simulink model "CicInterpolator75"  (Simulink 6.3)
settings: Solver=VariableStepDiscrete  SolverMode=SingleTasking  StartTime=0.0  StopTime=7000  FixedStep=1  RelTol=1e-3
InitFcn:
  | %% DSPBuilder Start
  | alt_dspbuilder_update_model(bdroot)
  | %% DSPBuilder End
libraries: allblocks_alteradspbuilder2 x15
settings Model: Creator=mjervis  LastModifiedBy=LKONG
settings DataIOCC: SignalLoggingName=sigsOut
settings OptimizationCC: BooleanDataType=off  InlineInvariantSignals=on
settings DebuggingCC: SolverPrmCheckMsg=none
settings HardwareCC: TargetUnknown=on

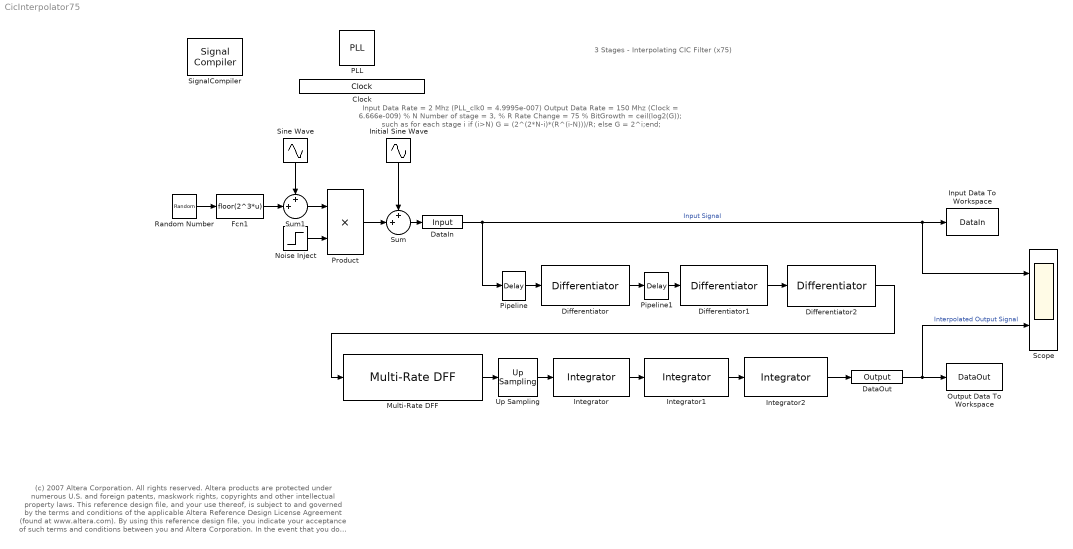
== system CicInterpolator75 ==
  note: 3 Stages - Interpolating CIC Filter (x75)
  note: (c) 2007 Altera Corporation. All rights reserved.  Altera products are protected under numerous U.S. and foreign patents, maskwork rights, copyrights and other intellectual property laws.
      | This reference design file, and your use thereof, is subject to and governed by the terms and conditions of the applicable Altera Reference Design License Agreement (found at www.altera.com).
      | By using this reference design file, you indicate your acceptance of such terms and conditions between you and Altera Corporation.
      | In the event that you do not agree with such terms and conditions, you may not use the reference design file and please promptly destroy any copies you have made.
      | This reference design file being provided on an "as-is" basis and as an accommodation and therefore all warranties, representations or guarantees of any kind (whether express, implied or statutory)
      | including, without limitation, warranties of merchantability, non-infringement, or fitness for a particular purpose, are specifically disclaimed.
      | By making this reference design file available, Altera expressly does not recommend, suggest or require that this reference design file be used in combination with any other product not provided by Altera
  note: Input Data Rate    = 2 Mhz (PLL_clk0 = 4.9995e-007)
      | Output Data Rate = 150 Mhz (Clock   = 6.666e-009)
      |
      | % N Number of stage = 3,
      | % R Rate Change = 75
      | % BitGrowth = ceil(log2(G)); such as for each stage i
      |      if (i>N)     G = (2^(2*N-i)*(R^(i-N)))/R;
      |      else         G = 2^i;end;
  Clock : allblocks_alteradspbuilder2/Clock  ClockPeriod=20/3  ClockPeriodUnit=ns  SampleTime=1  SimulationStartCycle=5  PhaseOffset=0  Reset=aclr  ResetType=Active Low  Export=off
  DataIn : allblocks_alteradspbuilder2/Input  iofile=d:\wsTrunk\workspace\Documentation\DesignExamples\Demos\Filters\CicFilter\Interpolator\tb_CicInterpolator75\CicInterpolator75_DataIn.salt  BusType=Signed Integer  bwl=8  bwr=0  SpecifyClock=on  clock=PLL_clk0  PORTTYPE=Input
  DataOut : allblocks_alteradspbuilder2/Output  iofile=d:\wsTrunk\workspace\Documentation\DesignExamples\Demos\Filters\CicFilter\Interpolator\tb_CicInterpolator75\CicInterpolator75_DataOut.capture  BusType=Signed Integer  bwl=29  bwr=0  PORTTYPE=Output
  Differentiator : allblocks_alteradspbuilder2/Differentiator  bwl=29  depth=1  use_ena=off  use_sclr=off
  Differentiator1 : allblocks_alteradspbuilder2/Differentiator  bwl=29  depth=1  use_ena=off  use_sclr=off
  Differentiator2 : allblocks_alteradspbuilder2/Differentiator  bwl=29  depth=1  use_ena=off  use_sclr=off
  Fcn1 : Fcn  Expr=floor(2^3*u)
  Initial Sine Wave : Sin  Orientation=down  SineType=Sample based  Amplitude=2^6 -1  SampleTime=75
  Input Data To Workspace : ToWorkspace  VariableName=DataIn  SampleTime=-1  SaveFormat=Array
  Integrator : allblocks_alteradspbuilder2/Integrator  bwl=29  depth=1  use_ena=off  use_sclr=off
  Integrator1 : allblocks_alteradspbuilder2/Integrator  bwl=29  depth=1  use_ena=off  use_sclr=off
  Integrator2 : allblocks_alteradspbuilder2/Integrator  bwl=29  depth=1  use_ena=off  use_sclr=off
  Multi-Rate DFF : allblocks_alteradspbuilder2/Multi-Rate DFF  pipeline=1  UseBaseClock=off  clock=Clock  use_ena=off  use_sclr=off
  Noise Inject : Step  Time=2500  SampleTime=75
  Output Data To Workspace : ToWorkspace  VariableName=DataOut  SampleTime=-1  SaveFormat=Array
  PLL : allblocks_alteradspbuilder2/PLL  clock_mult=[75, 75, 3, 4, 1, 1, 1, 1, 1]  clock_divide=[1, 1, 3, 1, 1, 1, 1, 1, 1]  clock_export=[0, 0, 0, 0, 0, 0, 0, 0, 0]  num_clocks=1  input_clock=Clock  use_base_clock=on
  Pipeline : allblocks_alteradspbuilder2/Delay  pipeline=1  ClockPhase=1  use_ena=off  use_sclr=off  use_init=off  reset_value=1
  Pipeline1 : allblocks_alteradspbuilder2/Delay  pipeline=1  ClockPhase=1  use_ena=off  use_sclr=off  use_init=off  reset_value=1
  Product : Product  SaturateOnIntegerOverflow=on  InputSameDT=on
  Random Number : RandomNumber  Variance=8  SampleTime=75
  Scope : Scope  NumInputPorts=2
      settings: TimeRange=7000  YMin=-100~-600000  YMax=150~600000  MaxDataPoints=10000
  SignalCompiler : allblocks_alteradspbuilder2/Signal Compiler  DeviceFamily=Stratix III  DeviceName=AUTO  EnableSignalTap=off  SignalTapDepth=128  UseBoardBlock=off  StpUseDefaultClock=on  StpClock=clock
  Sine Wave : Sin  Orientation=down  SineType=Sample based  Amplitude=2^3 -1  Samples=500  SampleTime=75
  Sum : Sum  Inputs=++|  SaturateOnIntegerOverflow=on  InputSameDT=on
  Sum1 : Sum  Inputs=++|  SaturateOnIntegerOverflow=on  InputSameDT=on
  Up Sampling : allblocks_alteradspbuilder2/Up Sampling  rate=75
  wires:
  Random Number/1 -> Fcn1/1
  Multi-Rate DFF/1 -> Up Sampling/1
  Differentiator/1 -> Pipeline1/1
  Integrator/1 -> Integrator1/1
  DataIn/1 -> Pipeline/1, Scope/1, Input Data To Workspace/1  "Input Signal"
  Differentiator1/1 -> Differentiator2/1
  Integrator1/1 -> Integrator2/1
  Integrator2/1 -> DataOut/1
  Sum/1 -> DataIn/1
  Noise Inject/1 -> Product/2
  Sum1/1 -> Product/1
  Differentiator2/1 -> Multi-Rate DFF/1
  DataOut/1 -> Scope/2, Output Data To Workspace/1  "Interpolated Output Signal"
  Pipeline/1 -> Differentiator/1
  Pipeline1/1 -> Differentiator1/1
  Up Sampling/1 -> Integrator/1
  Sine Wave/1 -> Sum1/1
  Fcn1/1 -> Sum1/2
  Initial Sine Wave/1 -> Sum/1
  Product/1 -> Sum/2
